simulink model "Simulation"  (R2018a)
settings: Solver=VariableStepAuto  StartTime=0.0  StopTime=50  RelTol=1e-3
values from neighbouring files (symbols this model uses):
  pitch_amp = pi/6    (= 0.523598775598)    [lqr_controller.m]
  pitch_freq = 0.4    [lqr_controller.m]
  yaw_amp = pi/4    (= 0.785398163397)    [lqr_controller.m]
  yaw_freq = 0.5    [lqr_controller.m]
libraries: cstblocks x18
settings Model: Creator=jobby246wc  LastModifiedBy=Student
settings CodeAppCC: StateflowObjectComments=on

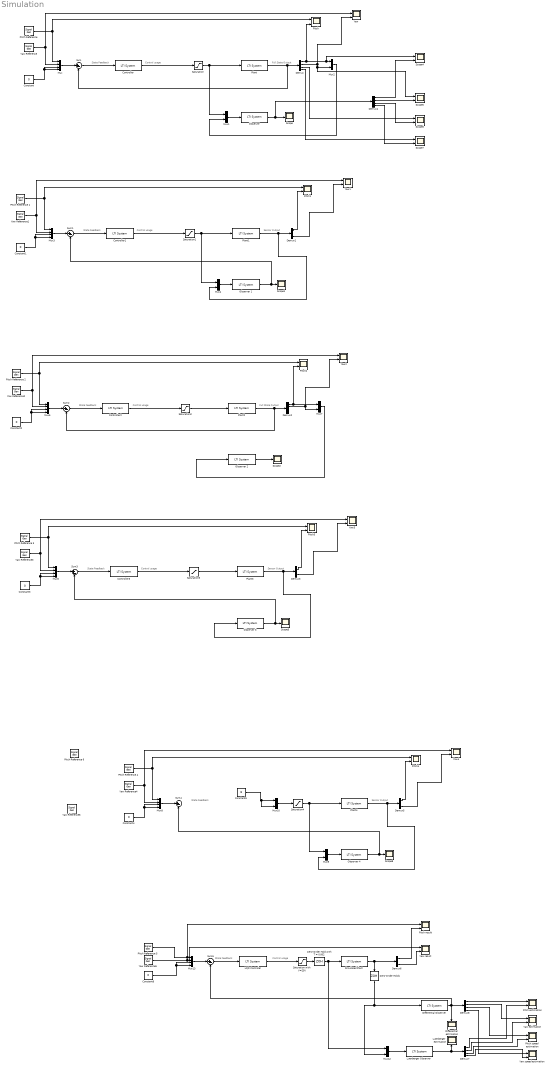
== system Simulation ==
  note: Full State Output
  note: State Feedback
  note: Control usage
  note: Control usage
  note: State Feedback
  note: Sensor Output
  note: Control usage
  note: State Feedback
  note: Full State Output
  note: Control usage
  note: State Feedback
  note: Sensor Output
  note: Sensor Output
  note: State Feedback
  note: State Feedback
  note: Control usage
  Constant{,1..4,6} (6 alike) : Constant  Value=0
  Constant5 : Constant  Value=8
  Controller{,1..3} (4 alike) : cstblocks/LTI System  sys=K  IC=[]
  Demux{,2,4,7..8} (5 alike) : Demux
  Demux{1,3,5..6} (4 alike) : Demux  Outputs=2
  Differential estimation : Scope
  Differential Observer : cstblocks/LTI System  sys=obs_sys_diff  IC=[]
  LQR Controler : cstblocks/LTI System  sys=K  IC=[]
  Luenberger estimation : Scope
  Luenberger Observer : cstblocks/LTI System  sys=obs_sys_luenberger  IC=[0,0,0,0]
  Mux{,3,5..6,8,13} (6 alike) : Mux
  Mux{1..2,4,7,9..10,12} (7 alike) : Mux  Inputs=2
  "Observer " : cstblocks/LTI System  sys=obs_sys_kalman  IC=[0,0,0,0]
  Observer 1 : cstblocks/LTI System  sys=obs_sys_kalman  IC=[0.1,0.1,0,0]
  Observer 2 : cstblocks/LTI System  sys=obs_sys_diff  IC=[]
  Observer 3 : cstblocks/LTI System  sys=obs_sys_diff  IC=[]
  Observer 4 : cstblocks/LTI System  sys=obs_sys_kalman  IC=[0,0,0,0]
  Pitch{,1..4} (5 alike) : Scope  NumInputPorts=2
  Pitch Reference {,1..5} (6 alike) : SignalGenerator  WaveForm=square  Amplitude=pitch_amp  Frequency=pitch_freq  Units=rad/sec
  Pitch Reference 6 : SignalGenerator  WaveForm=square  Amplitude=0  Frequency=pitch_freq  Units=rad/sec
  Pitch estimation : Scope  NumInputPorts=2
  Pitch result : Scope  NumInputPorts=2
  Pitch speed estimation : Scope  NumInputPorts=2
  Plant : cstblocks/LTI System  sys=control_sys  IC=[0.1,0.1,0,0]
  Plant1 : cstblocks/LTI System  sys=real_sys  IC=[0.1,0.1,0,0]
  Plant2 : cstblocks/LTI System  sys=control_sys  IC=[0.1,0.1,0,0]
  Plant3 : cstblocks/LTI System  sys=real_sys  IC=[0.1,0.1,0,0]
  Plant4 : cstblocks/LTI System  sys=real_sys  IC=[0.1,0.1,0,0]
  Saturation{,1..4} (5 alike) : Saturate  UpperLimit=25  LowerLimit=-25
  Saturation with V=25V : Saturate  UpperLimit=25  LowerLimit=-25
  Scope{,1..3,8} (5 alike) : Scope
  Scope{4..7} (4 alike) : Scope  NumInputPorts=2
  Simulated Plant : cstblocks/LTI System  sys=real_sys  IC=[0.1,0.1,0,0]
  Sum{,1..5} (6 alike) : Sum  Inputs=|+-
  Yaw{,1..4} (5 alike) : Scope  NumInputPorts=2
  Yaw Reference{,1..5} (6 alike) : SignalGenerator  WaveForm=square  Amplitude=yaw_amp  Frequency=yaw_freq  Units=rad/sec
  Yaw Reference6 : SignalGenerator  WaveForm=square  Amplitude=pi/3  Frequency=.1
  Yaw estimation : Scope  NumInputPorts=2
  Yaw result : Scope  NumInputPorts=2
  Yaw speed estimation : Scope  NumInputPorts=2
  Zero-Order Hold with T = 0.002 : ZeroOrderHold  SampleTime=0.002
  Zero-Order Hold1 : ZeroOrderHold  SampleTime=0.002
  wires:
  Plant/1 -> Demux/1, Sum/2
  Demux/1 -> Scope4/1, Mux2/1, Pitch/2
  Demux/2 -> Yaw/2, Scope5/1, Mux2/2
  Mux/1 -> Sum/1
  Sum/1 -> Controller/1
  "Pitch Reference "/1 -> Pitch/1, Mux/1
  Constant/1 -> Mux/3, Mux/4
  Yaw Reference/1 -> Mux/2, Yaw/1
  Saturation/1 -> Mux1/1, Plant/1
  Controller/1 -> Saturation/1
  Mux1/1 -> "Observer "/1
  Mux2/1 -> Mux1/2
  "Observer "/1 -> Demux4/1, Scope/1
  Demux1/2 -> Yaw1/2
  Constant1/1 -> Mux3/3, Mux3/4
  Mux3/1 -> Sum1/1
  Demux1/1 -> Pitch1/2
  Controller1/1 -> Saturation1/1
  Pitch Reference 1/1 -> Pitch1/1, Mux3/1
  Plant1/1 -> Demux1/1, Mux4/2
  Sum1/1 -> Controller1/1
  Saturation1/1 -> Mux4/1, Plant1/1
  Observer 1/1 -> Sum1/2, Scope1/1
  Yaw Reference1/1 -> Mux3/2, Yaw1/1
  Mux4/1 -> Observer 1/1
  Demux2/2 -> Yaw2/2, Mux7/2
  Constant2/1 -> Mux5/3, Mux5/4
  Mux5/1 -> Sum2/1
  Demux2/1 -> Mux7/1, Pitch2/2
  Controller2/1 -> Saturation2/1
  Pitch Reference 2/1 -> Pitch2/1, Mux5/1
  Plant2/1 -> Demux2/1, Sum2/2
  Sum2/1 -> Controller2/1
  Saturation2/1 -> Plant2/1
  Observer 2/1 -> Scope2/1
  Yaw Reference2/1 -> Mux5/2, Yaw2/1
  Mux7/1 -> Observer 2/1
  Sum3/1 -> Controller3/1
  Constant3/1 -> Mux6/3, Mux6/4
  Controller3/1 -> Saturation3/1
  Observer 3/1 -> Sum3/2, Scope3/1
  Pitch Reference 3/1 -> Pitch3/1, Mux6/1
  Demux3/1 -> Pitch3/2
  Mux6/1 -> Sum3/1
  Saturation3/1 -> Plant3/1
  Demux3/2 -> Yaw3/2
  Plant3/1 -> Observer 3/1, Demux3/1
  Yaw Reference3/1 -> Mux6/2, Yaw3/1
  Demux4/1 -> Scope4/2
  Demux4/2 -> Scope5/2
  Demux4/3 -> Scope6/2
  Demux/3 -> Scope6/1
  Demux4/4 -> Scope7/2
  Demux/4 -> Scope7/1
  Pitch Reference 4/1 -> Pitch4/1, Mux8/1
  Mux8/1 -> Sum4/1
  Constant4/1 -> Mux8/3, Mux8/4
  Yaw Reference4/1 -> Mux8/2, Yaw4/1
  Saturation4/1 -> Mux9/1, Plant4/1
  Mux9/1 -> Observer 4/1
  Observer 4/1 -> Sum4/2, Scope8/1
  Plant4/1 -> Demux5/1, Mux9/2
  Demux5/1 -> Pitch4/2
  Demux5/2 -> Yaw4/2
  Mux10/1 -> Saturation4/1
  Constant5/1 -> Mux10/2, Mux10/1
  Mux12/1 -> Luenberger Observer/1
  Mux13/1 -> Sum5/1
  Sum5/1 -> LQR Controler/1
  Saturation with V=25V/1 -> Zero-Order Hold with T = 0.002/1
  Constant6/1 -> Mux13/3, Mux13/4
  Yaw Reference5/1 -> Yaw result/1, Mux13/2
  Demux6/2 -> Yaw result/2
  Pitch Reference 5/1 -> Pitch result/1, Mux13/1
  Demux6/1 -> Pitch result/2
  Demux7/2 -> Yaw estimation/2
  Demux7/3 -> Pitch speed estimation/2
  Demux8/3 -> Pitch speed estimation/1
  Demux8/4 -> Yaw speed estimation/1
  Demux8/1 -> Pitch estimation/1
  Luenberger Observer/1 -> Demux7/1, Luenberger estimation/1
  Differential Observer/1 -> Differential estimation/1, Demux8/1, Sum5/2
  Demux7/4 -> Yaw speed estimation/2
  Demux7/1 -> Pitch estimation/2
  Demux8/2 -> Yaw estimation/1
  Simulated Plant/1 -> Demux6/1, Zero-Order Hold1/1
  Zero-Order Hold with T = 0.002/1 -> Simulated Plant/1, Mux12/1
  Zero-Order Hold1/1 -> Mux12/2, Differential Observer/1
  LQR Controler/1 -> Saturation with V=25V/1
